simulink model "DVS2X_All"  (R2021b)
settings: Solver=VariableStepAuto  StartTime=0.0  StopTime=0.1  RelTol=1e-3
values from neighbouring files (symbols this model uses):
  k1 = 10^(gain/10)    (= 3.16227766017)    [LNA_tests.m]
  k3 = -4/3*(k1/vip3^2)    [LNA_tests.m]
  k5 = -(0.10875*k1+(3/4)*(vp1dB^2))*((8/5)*(1/vp1dB^4))    [LNA_tests.m]
  vip3 = sqrt(2*10^((IIP3-30)/10)*R)    [LNA_tests.m]
undefined symbols (not defined in the file or in its folder): dvbsapskmod
libraries: commutil2 x23, commdigbbndapm x20, dspsrcs4 x20, commfilt2 x20, commrflib2 x14, commchan3 x12, commsink2 x10, commrandsrc3 x10, commrfcorlib x7, commeq3 x5
(part 1 of 2)
settings Model: SimulationMode=accelerator  Creator=Martha Ca$h  LastModifiedBy=Martha Ca$h
settings SolverCC: AlgebraicLoopSolver=TrustRegion
settings DebuggingCC: SFMachineParentedDataDiag=warning

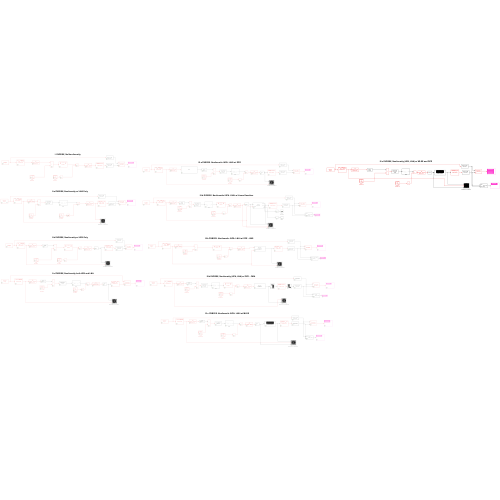
[thumbnail: Simulink's stored preview of the top-level diagram]
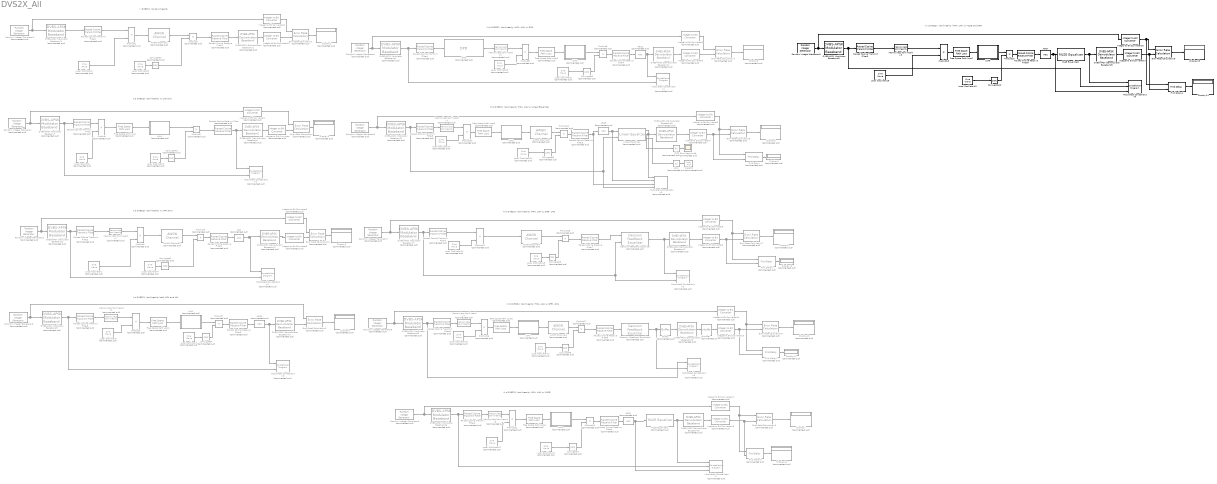
== system DVS2X_All ==
  note: I. DVB2SX, No Non-linearity
  note: II.a DVB2SX, Nonlinearity w/ LNA Only
  note: II.b DVB2SX, Nonlinearity w/ HPA Only
  note: Av
  note: II.c DVB2SX, Nonlinearity both HPA and LNA
  note: III.a DVB2SX, Nonlinearity (HPA, LNA) w/ DPD
  note: III.b DVB2SX, Nonlinearity (HPA, LNA) w/ Linear Equalizer
  note: III.c DVB2SX, Nonlinearity (HPA, LNA) w/ MLSE
  note: III.b DVB2SX, Nonlinearity (HPA, LNA) w/ DFE - LMS
  note: III.b DVB2SX, Nonlinearity (HPA, LNA) w/ DFE - CMA
  note: III.c DVB2SX, Nonlinearity (HPA, LNA) w/ MLSE and DPD
  AGC{,1..4} (5 alike) : commrfcorlib/AGC  Commented=on  LegacyMode=off  DetectorMethod=Rectifier  LoopMethod=Linear  UpdatePeriod=100  StepSize=0.1  AdaptationStepSize=0.01  DesiredOutputPower=1  AveragingLength=256  MaximumGain=30  MaxPowerGain=400  GainOutputPort=off  InputPowerOutputPort=off  SimulateUsing=Code generation
  AGC7 : commrfcorlib/AGC  LegacyMode=off  DetectorMethod=Rectifier  LoopMethod=Linear  UpdatePeriod=100  StepSize=0.1  AdaptationStepSize=0.01  DesiredOutputPower=1  AveragingLength=256  MaximumGain=30  MaxPowerGain=400  GainOutputPort=off  InputPowerOutputPort=off  SimulateUsing=Code generation
  AWGN Channel1 : commchan3/AWGN Channel  Commented=on  InputProcessing=Columns as channels (frame based)  seed=67  noiseMode="Signal to noise ratio  (Eb/No)"  EbNodB=0  EsNodB=10  SNRdB=10  bitsPerSym=4  Ps=1  Tsym=1e-6  variance=1
  AWGN Channel2 : commchan3/AWGN Channel  Commented=on  InputProcessing=Columns as channels (frame based)  seed=67  noiseMode="Signal to noise ratio  (Eb/No)"  EbNodB=23  EsNodB=10  SNRdB=10  bitsPerSym=4  Ps=1  Tsym=1e-6  variance=1
  AWGN Channel3 : commchan3/AWGN Channel  Commented=on  InputProcessing=Columns as channels (frame based)  seed=67  noiseMode="Signal to noise ratio  (Eb/No)"  EbNodB=50  EsNodB=10  SNRdB=10  bitsPerSym=4  Ps=1  Tsym=1e-6  variance=1
  AWGN Channel4 : commchan3/AWGN Channel  Commented=on  InputProcessing=Columns as channels (frame based)  seed=67  noiseMode="Signal to noise ratio  (Eb/No)"  EbNodB=23  EsNodB=10  SNRdB=10  bitsPerSym=4  Ps=1  Tsym=1e-6  variance=1
  AWGN Channel5 : commchan3/AWGN Channel  Commented=on  InputProcessing=Columns as channels (frame based)  seed=67  noiseMode="Signal to noise ratio  (Eb/No)"  EbNodB=23  EsNodB=10  SNRdB=10  bitsPerSym=4  Ps=1  Tsym=1e-6  variance=1
  Abs1 : Abs  Commented=on
  Abs2 : Abs  Commented=on
  Buffer : Buffer  Commented=on  N=16  OutputFrames=off
  Conjugate{1..9} (9 alike) : Math  Commented=on  Operator=conj  SignedPower=on  SaturateOnIntegerOverflow=on
  Conjugate10 : Math  Operator=conj  SignedPower=on  SaturateOnIntegerOverflow=on
  DPD : commrfcorlib/DPD  Commented=on  PolynomialType=Memory polynomial  CoefficientSource=Property  Coefficients=complex([1 0 0 0 0; 0 0 0 0 0; 0 0 0 0 0])  SimulateUsing=Code generation
      settings: SourceProductBaseCode=CM
  DVBS-APSK Demodulator Baseband{,1..8} (9 alike) : commdigbbndapm/DVBS-APSK Demodulator Baseband  Commented=on  StdSuffix=S2  FrameLength=Normal  ModOrder=16  CodeIDF=2/3  NormalizationMethod=Outer radius as 1  OutputType=Integer  DecisionType=Hard decision  VarianceSource=Property  NoiseVariance=1  OutputDataType=double  SimulateUsing=Interpreted execution
      settings: SourceProductBaseCode=CM
  DVBS-APSK Demodulator Baseband9 : commdigbbndapm/DVBS-APSK Demodulator Baseband  StdSuffix=S2  FrameLength=Normal  ModOrder=16  CodeIDF=2/3  NormalizationMethod=Outer radius as 1  OutputType=Integer  DecisionType=Hard decision  VarianceSource=Property  NoiseVariance=1  OutputDataType=double  SimulateUsing=Interpreted execution
      settings: SourceProductBaseCode=CM
  DVBS-APSK Modulator Baseband{,1..8} (9 alike) : commdigbbndapm/DVBS-APSK Modulator Baseband  Commented=on  StdSuffix=S2  FrameLength=Normal  ModOrder=16  CodeIDF=2/3  NormalizationMethod=Outer radius as 1  InputType=Integer  OutputDataType=double  SimulateUsing=Code generation
      settings: SourceProductBaseCode=CM
  DVBS-APSK Modulator Baseband9 : commdigbbndapm/DVBS-APSK Modulator Baseband  StdSuffix=S2  FrameLength=Normal  ModOrder=16  CodeIDF=2/3  NormalizationMethod=Outer radius as 1  InputType=Integer  OutputDataType=double  SimulateUsing=Code generation
      settings: SourceProductBaseCode=CM
  Decision Feedback Equalizer : commeq3/Decision Feedback Equalizer  Commented=on  NumForwardTaps=5  NumFeedbackTaps=3  Constellation=dvbsapskmod(0:15, 16, 's2', '2/3')  InputSamplesPerSymbol=1  Algorithm=LMS  StepSize=0.01  ForgettingFactor=0.99  InitialInverseCorrelationMatrix=0.1  ReferenceTap=3  InputDelay=0  AdaptWeightsSource=Property  AdaptWeights=on  InitialWeightsSource=Auto  InitialWeights=0  TrainingInitialWeights=0  BlindInitialWeights=[ 0; 0; 1; 0; 0; 0; 0; 0 ]  WeightUpdatePeriod=1  TrainingFlagInputPort=off  AdaptAfterTraining=on  ResetInputPort=off  ErrorOutputPort=off  TapWeightsOutputPort=off  SimulateUsing=Code generation
      settings: SourceProductBaseCode=CM
  Decision Feedback Equalizer1 : commeq3/Decision Feedback Equalizer  Commented=on  NumForwardTaps=5  NumFeedbackTaps=3  Constellation=dvbsapskmod(0:15, 16, 's2', '2/3')  InputSamplesPerSymbol=1  Algorithm=CMA  StepSize=0.01  ForgettingFactor=0.99  InitialInverseCorrelationMatrix=0.1  ReferenceTap=3  InputDelay=0  AdaptWeightsSource=Property  AdaptWeights=on  InitialWeightsSource=Auto  InitialWeights=0  TrainingInitialWeights=0  BlindInitialWeights=[ 0; 0; 1; 0; 0; 0; 0; 0 ]  WeightUpdatePeriod=1  TrainingFlagInputPort=off  AdaptAfterTraining=on  ResetInputPort=off  ErrorOutputPort=off  TapWeightsOutputPort=off  SimulateUsing=Code generation
      settings: SourceProductBaseCode=CM
  Display{1..13} (13 alike) : Display  Commented=on
  Display14 : Display
  Display15 : Display
  Error Magnitude : Scope  Commented=on
  Error Rate Calculation : commsink2/Error Rate Calculation  Commented=on  N=40  st_delay=150  cp_mode=Entire frame  subframe=[]  PMode=Port  WsName=ErrorVec1  RsMode2=off  stop=off  numErr=100  maxBits=1e6
  Error Rate Calculation1 : commsink2/Error Rate Calculation  Commented=on  N=40  st_delay=0  cp_mode=Entire frame  subframe=[]  PMode=Port  WsName=ErrorVec1  RsMode2=off  stop=off  numErr=100  maxBits=1e6
  Error Rate Calculation2 : commsink2/Error Rate Calculation  Commented=on  N=40  st_delay=0  cp_mode=Entire frame  subframe=[]  PMode=Port  WsName=ErrorVec1  RsMode2=off  stop=off  numErr=100  maxBits=1e6
  Error Rate Calculation3 : commsink2/Error Rate Calculation  Commented=on  N=10  st_delay=0  cp_mode=Entire frame  subframe=[]  PMode=Port  WsName=ErrorVec1  RsMode2=off  stop=off  numErr=100  maxBits=1e6
  Error Rate Calculation4 : commsink2/Error Rate Calculation  Commented=on  N=40  st_delay=0  cp_mode=Entire frame  subframe=[]  PMode=Port  WsName=ErrorVec1  RsMode2=off  stop=off  numErr=100  maxBits=1e6
  Error Rate Calculation5 : commsink2/Error Rate Calculation  Commented=on  N=40  st_delay=10000  cp_mode=Entire frame  subframe=[]  PMode=Port  WsName=ErrorVec1  RsMode2=off  stop=off  numErr=100  maxBits=1e6
  Error Rate Calculation6 : commsink2/Error Rate Calculation  Commented=on  N=80  st_delay=0  cp_mode=Entire frame  subframe=[]  PMode=Port  WsName=ErrorVec1  RsMode2=off  stop=off  numErr=100  maxBits=1e6
  Error Rate Calculation7 : commsink2/Error Rate Calculation  Commented=on  N=53  st_delay=10000  cp_mode=Entire frame  subframe=[]  PMode=Port  WsName=ErrorVec1  RsMode2=off  stop=off  numErr=100  maxBits=1e6
  Error Rate Calculation8 : commsink2/Error Rate Calculation  Commented=on  N=40  st_delay=10000  cp_mode=Entire frame  subframe=[]  PMode=Port  WsName=ErrorVec1  RsMode2=off  stop=off  numErr=100  maxBits=1e6
  Error Rate Calculation9 : commsink2/Error Rate Calculation  N=80  st_delay=400  cp_mode=Entire frame  subframe=[]  PMode=Port  WsName=ErrorVec1  RsMode2=off  stop=off  numErr=100  maxBits=1e6
  Find Delay : commutil2/Find Delay  Commented=on  corrLength=10000  chgSigOP=off  stopUpdate=off  numConstDelay=3
      settings: SourceProductBaseCode=CM
  Find Delay1 : commutil2/Find Delay  Commented=on  corrLength=10000  chgSigOP=off  stopUpdate=off  numConstDelay=3
      settings: SourceProductBaseCode=CM
  Find Delay2 : commutil2/Find Delay  Commented=on  corrLength=10000  chgSigOP=off  stopUpdate=off  numConstDelay=3
      settings: SourceProductBaseCode=CM
  Find Delay3 : commutil2/Find Delay  Commented=on  corrLength=1000  chgSigOP=off  stopUpdate=off  numConstDelay=3
      settings: SourceProductBaseCode=CM
  Find Delay4 : commutil2/Find Delay  corrLength=1000  chgSigOP=off  stopUpdate=off  numConstDelay=3
      settings: SourceProductBaseCode=CM
  Free Space Path Loss{,1..4,6} (6 alike) : commrflib2/Free Space Path Loss  Commented=on  mode=Decibels  dB=10  d=0.100  fc=1920
      settings: SourceProductBaseCode=CM
  Free Space Path Loss7 : commrflib2/Free Space Path Loss  mode=Decibels  dB=10  d=0.100  fc=1920
      settings: SourceProductBaseCode=CM
  Integer to Bit Converter{,1..15} (16 alike) : commutil2/Integer to Bit Converter  Commented=on  nbits=4  signedInputValues=Unsigned  bitOrder=MSB first  outDtype=Inherit via internal rule
  Integer to Bit Converter16 : commutil2/Integer to Bit Converter  nbits=4  signedInputValues=Unsigned  bitOrder=MSB first  outDtype=Inherit via internal rule
  Integer to Bit Converter17 : commutil2/Integer to Bit Converter  nbits=4  signedInputValues=Unsigned  bitOrder=MSB first  outDtype=Inherit via internal rule
  LNA1 : Subsystem  Commented=on
  LNA2 : Subsystem  Commented=on
  LNA3 : Subsystem  Commented=on
  LNA4 : Subsystem  Commented=on
  LNA5 : Subsystem  Commented=on
  LNA7 : Subsystem  Commented=on
  LNA8 : Subsystem
  Linear Equalizer : commeq3/Linear Equalizer  Commented=on  NumTaps=5  Constellation=dvbsapskmod(0:15, 16, 's2', '2/3')  InputSamplesPerSymbol=1  Algorithm=LMS  StepSize=0.01  ForgettingFactor=0.99  InitialInverseCorrelationMatrix=0.1  ReferenceTap=3  InputDelay=0  AdaptWeightsSource=Property  AdaptWeights=on  InitialWeightsSource=Auto  InitialWeights=0  TrainingInitialWeights=0  BlindInitialWeights=[ 0; 0; 1; 0; 0 ]  WeightUpdatePeriod=1  TrainingFlagInputPort=off  AdaptAfterTraining=on  ResetInputPort=off  ErrorOutputPort=on  TapWeightsOutputPort=on  SimulateUsing=Interpreted execution
      settings: SourceProductBaseCode=CM
  Local Oscillator{,1..17} (18 alike) : dspsrcs4/Sine Wave  Commented=on  Amplitude=1  Frequency=1.5e9  Phase=0  SampleMode=Discrete  OutComplex=Complex  CompMethod=Trigonometric fcn  TableSize=Speed  SampleTime=(1e-6)/8  SamplesPerFrame=8  ResetState=Restart at time zero  OutputFrames=off  dataType=double  wordLen=16  udDataType=sfix(16)  fracBitsMode=Best precision  numFracBits=15  OutDataTypeStr=double  LastOutDataTypeStr=double
  Local Oscillator18 : dspsrcs4/Sine Wave  Amplitude=1  Frequency=1.5e9  Phase=0  SampleMode=Discrete  OutComplex=Complex  CompMethod=Trigonometric fcn  TableSize=Speed  SampleTime=(1e-6)/8  SamplesPerFrame=8  ResetState=Restart at time zero  OutputFrames=off  dataType=double  wordLen=16  udDataType=sfix(16)  fracBitsMode=Best precision  numFracBits=15  OutDataTypeStr=double  LastOutDataTypeStr=double
  Local Oscillator19 : dspsrcs4/Sine Wave  Amplitude=1  Frequency=1.5e9  Phase=0  SampleMode=Discrete  OutComplex=Complex  CompMethod=Trigonometric fcn  TableSize=Speed  SampleTime=(1e-6)/8  SamplesPerFrame=8  ResetState=Restart at time zero  OutputFrames=off  dataType=double  wordLen=16  udDataType=sfix(16)  fracBitsMode=Best precision  numFracBits=15  OutDataTypeStr=double  LastOutDataTypeStr=double
  MLSE Equalizer1 : commeq3/MLSE Equalizer  Commented=on  specchan=Dialog  chancoeff=1  constpts=dvbsapskmod(0:15, 16, 's2', '2/3')  tbdepth=10  opmode=Continuous with reset option  enpreamble=off  preamble=[0 3 2 1]  enpostamble=off  postamble=[0 2 3 1]  numsamp=1  reset=off
      settings: SourceProductBaseCode=CM
  MLSE Equalizer2 : commeq3/MLSE Equalizer  specchan=Dialog  chancoeff=1  constpts=dvbsapskmod(0:15, 16, 's2', '2/3')  tbdepth=10  opmode=Continuous with reset option  enpreamble=off  preamble=[0 3 2 1]  enpostamble=off  postamble=[0 2 3 1]  numsamp=1  reset=off
      settings: SourceProductBaseCode=CM
  Memoryless Nonlinearity1 : commrflib2/Memoryless Nonlinearity  Commented=on  model_select=Saleh model  linGaindB=0  GindB=GindB  iip3=30  am2pm=10  LPwrLimAMPM=10  UPwrLimAMPM=inf  amam=[2.1587 1.1517]  ampm=[4.0330 9.1040]  x=[8.1081 1.5413 6.5202 -0.0718]  y=[4.6645 2.0965 10.88 -0.003]  p=0.5  GoutdB=GoutdB  vsat=1
      settings: SourceProductBaseCode=CM
  Memoryless Nonlinearity2 : commrflib2/Memoryless Nonlinearity  Commented=on  model_select=Saleh model  linGaindB=0  GindB=GindB  iip3=30  am2pm=10  LPwrLimAMPM=10  UPwrLimAMPM=inf  amam=[2.1587 1.1517]  ampm=[4.0330 9.1040]  x=[8.1081 1.5413 6.5202 -0.0718]  y=[4.6645 2.0965 10.88 -0.003]  p=0.5  GoutdB=GoutdB  vsat=1
      settings: SourceProductBaseCode=CM
  Memoryless Nonlinearity3 : commrflib2/Memoryless Nonlinearity  Commented=on  model_select=Saleh model  linGaindB=0  GindB=GindB  iip3=30  am2pm=10  LPwrLimAMPM=10  UPwrLimAMPM=inf  amam=[2.1587 1.1517]  ampm=[4.0330 9.1040]  x=[8.1081 1.5413 6.5202 -0.0718]  y=[4.6645 2.0965 10.88 -0.003]  p=0.5  GoutdB=GoutdB  vsat=1
      settings: SourceProductBaseCode=CM
  Memoryless Nonlinearity4 : commrflib2/Memoryless Nonlinearity  Commented=on  model_select=Saleh model  linGaindB=0  GindB=-7.626571802255640  iip3=30  am2pm=10  LPwrLimAMPM=10  UPwrLimAMPM=inf  amam=[2.1587 1.1517]  ampm=[4.0330 9.1040]  x=[8.1081 1.5413 6.5202 -0.0718]  y=[4.6645 2.0965 10.88 -0.003]  p=0.5  GoutdB=9.911826101838730  vsat=1
      settings: SourceProductBaseCode=CM
  Memoryless Nonlinearity5 : commrflib2/Memoryless Nonlinearity  Commented=on  model_select=Saleh model  linGaindB=0  GindB=-7.626571802255640  iip3=30  am2pm=10  LPwrLimAMPM=10  UPwrLimAMPM=inf  amam=[2.1587 1.1517]  ampm=[4.0330 9.1040]  x=[8.1081 1.5413 6.5202 -0.0718]  y=[4.6645 2.0965 10.88 -0.003]  p=0.5  GoutdB=9.911826101838730  vsat=1
      settings: SourceProductBaseCode=CM
  Memoryless Nonlinearity7 : commrflib2/Memoryless Nonlinearity  Commented=on  model_select=Saleh model  linGaindB=0  GindB=-7.626571802255640  iip3=30  am2pm=10  LPwrLimAMPM=10  UPwrLimAMPM=inf  amam=[2.1587 1.1517]  ampm=[4.0330 9.1040]  x=[8.1081 1.5413 6.5202 -0.0718]  y=[4.6645 2.0965 10.88 -0.003]  p=0.5  GoutdB=9.911826101838730  vsat=1
      settings: SourceProductBaseCode=CM
  Memoryless Nonlinearity8 : commrflib2/Memoryless Nonlinearity  model_select=Saleh model  linGaindB=0  GindB=-7.626571802255640  iip3=30  am2pm=10  LPwrLimAMPM=10  UPwrLimAMPM=inf  amam=[2.1587 1.1517]  ampm=[4.0330 9.1040]  x=[8.1081 1.5413 6.5202 -0.0718]  y=[4.6645 2.0965 10.88 -0.003]  p=0.5  GoutdB=9.911826101838730  vsat=1
      settings: SourceProductBaseCode=CM
  Modulated Constellation{1..4,6,8} (6 alike) : ConstellationDiagram  Commented=on  NumInputPorts=2
  Modulated Constellation5 : ConstellationDiagram  Commented=on  NumInputPorts=4
  Modulated Constellation7 : ConstellationDiagram  Commented=on  NumInputPorts=3
  Modulated Constellation9 : ConstellationDiagram  NumInputPorts=3
  Product{,1..17} (18 alike) : Product  Commented=on
  Product18 : Product
  Product19 : Product
  Raised Cosine Receive Filter : commfilt2/Raised Cosine Receive Filter  Commented=on  filtType=Square root  R=0.2  filtSpan=10  N=8  downFactor=8  downOffset=0  filterGain=1  InputProcessing=Columns as channels (frame based)  RateOptions=Enforce single-rate processing  framing=Mute  checkCoeff=off  variableName=rcRxFilt  currentFiltSpan=10  D=(10)/2  inputOffset=0  sampMode=Mute  saveAsFlag=0  rateMode=Downsampling  checkGain=Normalized  launchFVT=on  roundingMode=Floor  overflowMode=off  coeffDataTypeStr=Inherit: Same word length as input  coeffMin=[]  coeffMax=[]  coeffLastDataTypeStr=Inherit: Same word length as input  accumDataTypeStr=Inherit: Same as product output  accumLastDataTypeStr=Inherit: Same as product output  outputDataTypeStr=Inherit: Same as accumulator  outputMin=[]  outputMax=[]  outputLastDataTypeStr=Inherit: Same as accumulator
  Raised Cosine Receive Filter1 : commfilt2/Raised Cosine Receive Filter  Commented=on  filtType=Square root  R=0.2  filtSpan=10  N=8  downFactor=8  downOffset=0  filterGain=1  InputProcessing=Columns as channels (frame based)  RateOptions=Enforce single-rate processing  framing=Mute  checkCoeff=off  variableName=rcRxFilt1  currentFiltSpan=10  D=(10)/2  inputOffset=0  sampMode=Mute  saveAsFlag=0  rateMode=Downsampling  checkGain=Normalized  launchFVT=on  roundingMode=Floor  overflowMode=off  coeffDataTypeStr=Inherit: Same word length as input  coeffMin=[]  coeffMax=[]  coeffLastDataTypeStr=Inherit: Same word length as input  accumDataTypeStr=Inherit: Same as product output  accumLastDataTypeStr=Inherit: Same as product output  outputDataTypeStr=Inherit: Same as accumulator  outputMin=[]  outputMax=[]  outputLastDataTypeStr=Inherit: Same as accumulator
  Raised Cosine Receive Filter2 : commfilt2/Raised Cosine Receive Filter  Commented=on  filtType=Square root  R=0.2  filtSpan=10  N=8  downFactor=8  downOffset=0  filterGain=1  InputProcessing=Columns as channels (frame based)  RateOptions=Enforce single-rate processing  framing=Mute  checkCoeff=off  variableName=rcRxFilt2  currentFiltSpan=10  D=(10)/2  inputOffset=0  sampMode=Mute  saveAsFlag=0  rateMode=Downsampling  checkGain=Normalized  launchFVT=on  roundingMode=Floor  overflowMode=off  coeffDataTypeStr=Inherit: Same word length as input  coeffMin=[]  coeffMax=[]  coeffLastDataTypeStr=Inherit: Same word length as input  accumDataTypeStr=Inherit: Same as product output  accumLastDataTypeStr=Inherit: Same as product output  outputDataTypeStr=Inherit: Same as accumulator  outputMin=[]  outputMax=[]  outputLastDataTypeStr=Inherit: Same as accumulator
  Raised Cosine Receive Filter3 : commfilt2/Raised Cosine Receive Filter  Commented=on  filtType=Square root  R=0.2  filtSpan=10  N=8  downFactor=8  downOffset=0  filterGain=1  InputProcessing=Columns as channels (frame based)  RateOptions=Enforce single-rate processing  framing=Mute  checkCoeff=off  variableName=rcRxFilt3  currentFiltSpan=10  D=(10)/2  inputOffset=0  sampMode=Mute  saveAsFlag=0  rateMode=Downsampling  checkGain=Normalized  launchFVT=on  roundingMode=Floor  overflowMode=off  coeffDataTypeStr=Inherit: Same word length as input  coeffMin=[]  coeffMax=[]  coeffLastDataTypeStr=Inherit: Same word length as input  accumDataTypeStr=Inherit: Same as product output  accumLastDataTypeStr=Inherit: Same as product output  outputDataTypeStr=Inherit: Same as accumulator  outputMin=[]  outputMax=[]  outputLastDataTypeStr=Inherit: Same as accumulator
  Raised Cosine Receive Filter4 : commfilt2/Raised Cosine Receive Filter  Commented=on  filtType=Square root  R=0.2  filtSpan=10  N=8  downFactor=8  downOffset=0  filterGain=1  InputProcessing=Columns as channels (frame based)  RateOptions=Enforce single-rate processing  framing=Mute  checkCoeff=off  variableName=rcRxFilt4  currentFiltSpan=10  D=(10)/2  inputOffset=0  sampMode=Mute  saveAsFlag=0  rateMode=Downsampling  checkGain=Normalized  launchFVT=on  roundingMode=Floor  overflowMode=off  coeffDataTypeStr=Inherit: Same word length as input  coeffMin=[]  coeffMax=[]  coeffLastDataTypeStr=Inherit: Same word length as input  accumDataTypeStr=Inherit: Same as product output  accumLastDataTypeStr=Inherit: Same as product output  outputDataTypeStr=Inherit: Same as accumulator  outputMin=[]  outputMax=[]  outputLastDataTypeStr=Inherit: Same as accumulator
  Raised Cosine Receive Filter5 : commfilt2/Raised Cosine Receive Filter  Commented=on  filtType=Square root  R=0.2  filtSpan=10  N=8  downFactor=8  downOffset=0  filterGain=1  InputProcessing=Columns as channels (frame based)  RateOptions=Enforce single-rate processing  framing=Mute  checkCoeff=off  variableName=rcRxFilt5  currentFiltSpan=10  D=(10)/2  inputOffset=0  sampMode=Mute  saveAsFlag=0  rateMode=Downsampling  checkGain=Normalized  launchFVT=on  roundingMode=Floor  overflowMode=off  coeffDataTypeStr=Inherit: Same word length as input  coeffMin=[]  coeffMax=[]  coeffLastDataTypeStr=Inherit: Same word length as input  accumDataTypeStr=Inherit: Same as product output  accumLastDataTypeStr=Inherit: Same as product output  outputDataTypeStr=Inherit: Same as accumulator  outputMin=[]  outputMax=[]  outputLastDataTypeStr=Inherit: Same as accumulator
  Raised Cosine Receive Filter6 : commfilt2/Raised Cosine Receive Filter  Commented=on  filtType=Square root  R=0.2  filtSpan=10  N=8  downFactor=8  downOffset=0  filterGain=1  InputProcessing=Columns as channels (frame based)  RateOptions=Enforce single-rate processing  framing=Mute  checkCoeff=off  variableName=rcRxFilt6  currentFiltSpan=10  D=(10)/2  inputOffset=0  sampMode=Mute  saveAsFlag=0  rateMode=Downsampling  checkGain=Normalized  launchFVT=on  roundingMode=Floor  overflowMode=off  coeffDataTypeStr=Inherit: Same word length as input  coeffMin=[]  coeffMax=[]  coeffLastDataTypeStr=Inherit: Same word length as input  accumDataTypeStr=Inherit: Same as product output  accumLastDataTypeStr=Inherit: Same as product output  outputDataTypeStr=Inherit: Same as accumulator  outputMin=[]  outputMax=[]  outputLastDataTypeStr=Inherit: Same as accumulator
  Raised Cosine Receive Filter7 : commfilt2/Raised Cosine Receive Filter  Commented=on  filtType=Square root  R=0.2  filtSpan=10  N=8  downFactor=8  downOffset=0  filterGain=1  InputProcessing=Columns as channels (frame based)  RateOptions=Enforce single-rate processing  framing=Mute  checkCoeff=off  variableName=rcRxFilt7  currentFiltSpan=10  D=(10)/2  inputOffset=0  sampMode=Mute  saveAsFlag=0  rateMode=Downsampling  checkGain=Normalized  launchFVT=on  roundingMode=Floor  overflowMode=off  coeffDataTypeStr=Inherit: Same word length as input  coeffMin=[]  coeffMax=[]  coeffLastDataTypeStr=Inherit: Same word length as input  accumDataTypeStr=Inherit: Same as product output  accumLastDataTypeStr=Inherit: Same as product output  outputDataTypeStr=Inherit: Same as accumulator  outputMin=[]  outputMax=[]  outputLastDataTypeStr=Inherit: Same as accumulator
  Raised Cosine Receive Filter8 : commfilt2/Raised Cosine Receive Filter  Commented=on  filtType=Square root  R=0.2  filtSpan=10  N=8  downFactor=8  downOffset=0  filterGain=1  InputProcessing=Columns as channels (frame based)  RateOptions=Enforce single-rate processing  framing=Mute  checkCoeff=off  variableName=rcRxFilt8  currentFiltSpan=10  D=(10)/2  inputOffset=0  sampMode=Mute  saveAsFlag=0  rateMode=Downsampling  checkGain=Normalized  launchFVT=on  roundingMode=Floor  overflowMode=off  coeffDataTypeStr=Inherit: Same word length as input  coeffMin=[]  coeffMax=[]  coeffLastDataTypeStr=Inherit: Same word length as input  accumDataTypeStr=Inherit: Same as product output  accumLastDataTypeStr=Inherit: Same as product output  outputDataTypeStr=Inherit: Same as accumulator  outputMin=[]  outputMax=[]  outputLastDataTypeStr=Inherit: Same as accumulator
  Raised Cosine Receive Filter9 : commfilt2/Raised Cosine Receive Filter  filtType=Square root  R=0.2  filtSpan=10  N=8  downFactor=8  downOffset=0  filterGain=1  InputProcessing=Columns as channels (frame based)  RateOptions=Enforce single-rate processing  framing=Mute  checkCoeff=off  variableName=rcRxFilt9  currentFiltSpan=10  D=(10)/2  inputOffset=0  sampMode=Mute  saveAsFlag=0  rateMode=Downsampling  checkGain=Normalized  launchFVT=on  roundingMode=Floor  overflowMode=off  coeffDataTypeStr=Inherit: Same word length as input  coeffMin=[]  coeffMax=[]  coeffLastDataTypeStr=Inherit: Same word length as input  accumDataTypeStr=Inherit: Same as product output  accumLastDataTypeStr=Inherit: Same as product output  outputDataTypeStr=Inherit: Same as accumulator  outputMin=[]  outputMax=[]  outputLastDataTypeStr=Inherit: Same as accumulator
  Raised Cosine Transmit Filter : commfilt2/Raised Cosine Transmit Filter  Commented=on  filtType=Square root  R=0.2  filtSpan=10  N=8  filterGain=1  InputProcessing=Columns as channels (frame based)  RateOptions=Enforce single-rate processing  framing=Mute  checkCoeff=on  variableName=rcTxFilt  checkGain=Normalized  sampMode=Mute  saveAsFlag=0  currentFiltSpan=10  D=(10)/2  launchFVT=on  roundingMode=Floor  overflowMode=off  coeffDataTypeStr=Inherit: Same word length as input  coeffMin=[]  coeffMax=[]  coeffLastDataTypeStr=Inherit: Same word length as input  outputDataTypeStr=Inherit: Same as accumulator  outputMin=[]  outputMax=[]  outputLastDataTypeStr=Inherit: Same as accumulator
  Raised Cosine Transmit Filter1 : commfilt2/Raised Cosine Transmit Filter  Commented=on  filtType=Square root  R=0.2  filtSpan=10  N=8  filterGain=1  InputProcessing=Columns as channels (frame based)  RateOptions=Enforce single-rate processing  framing=Mute  checkCoeff=on  variableName=rcTxFilt1  checkGain=Normalized  sampMode=Mute  saveAsFlag=0  currentFiltSpan=10  D=(10)/2  launchFVT=on  roundingMode=Floor  overflowMode=off  coeffDataTypeStr=Inherit: Same word length as input  coeffMin=[]  coeffMax=[]  coeffLastDataTypeStr=Inherit: Same word length as input  outputDataTypeStr=Inherit: Same as accumulator  outputMin=[]  outputMax=[]  outputLastDataTypeStr=Inherit: Same as accumulator
  Raised Cosine Transmit Filter2 : commfilt2/Raised Cosine Transmit Filter  Commented=on  filtType=Square root  R=0.2  filtSpan=10  N=8  filterGain=1  InputProcessing=Columns as channels (frame based)  RateOptions=Enforce single-rate processing  framing=Mute  checkCoeff=on  variableName=rcTxFilt2  checkGain=Normalized  sampMode=Mute  saveAsFlag=0  currentFiltSpan=10  D=(10)/2  launchFVT=on  roundingMode=Floor  overflowMode=off  coeffDataTypeStr=Inherit: Same word length as input  coeffMin=[]  coeffMax=[]  coeffLastDataTypeStr=Inherit: Same word length as input  outputDataTypeStr=Inherit: Same as accumulator  outputMin=[]  outputMax=[]  outputLastDataTypeStr=Inherit: Same as accumulator
  Raised Cosine Transmit Filter3 : commfilt2/Raised Cosine Transmit Filter  Commented=on  filtType=Square root  R=0.2  filtSpan=10  N=8  filterGain=1  InputProcessing=Columns as channels (frame based)  RateOptions=Enforce single-rate processing  framing=Mute  checkCoeff=on  variableName=rcTxFilt3  checkGain=Normalized  sampMode=Mute  saveAsFlag=0  currentFiltSpan=10  D=(10)/2  launchFVT=on  roundingMode=Floor  overflowMode=off  coeffDataTypeStr=Inherit: Same word length as input  coeffMin=[]  coeffMax=[]  coeffLastDataTypeStr=Inherit: Same word length as input  outputDataTypeStr=Inherit: Same as accumulator  outputMin=[]  outputMax=[]  outputLastDataTypeStr=Inherit: Same as accumulator
  Raised Cosine Transmit Filter4 : commfilt2/Raised Cosine Transmit Filter  Commented=on  filtType=Square root  R=0.2  filtSpan=10  N=8  filterGain=1  InputProcessing=Columns as channels (frame based)  RateOptions=Enforce single-rate processing  framing=Mute  checkCoeff=on  variableName=rcTxFilt4  checkGain=Normalized  sampMode=Mute  saveAsFlag=0  currentFiltSpan=10  D=(10)/2  launchFVT=on  roundingMode=Floor  overflowMode=off  coeffDataTypeStr=Inherit: Same word length as input  coeffMin=[]  coeffMax=[]  coeffLastDataTypeStr=Inherit: Same word length as input  outputDataTypeStr=Inherit: Same as accumulator  outputMin=[]  outputMax=[]  outputLastDataTypeStr=Inherit: Same as accumulator
  Raised Cosine Transmit Filter5 : commfilt2/Raised Cosine Transmit Filter  Commented=on  filtType=Square root  R=0.2  filtSpan=10  N=8  filterGain=1  InputProcessing=Columns as channels (frame based)  RateOptions=Enforce single-rate processing  framing=Mute  checkCoeff=on  variableName=rcTxFilt5  checkGain=Normalized  sampMode=Mute  saveAsFlag=0  currentFiltSpan=10  D=(10)/2  launchFVT=on  roundingMode=Floor  overflowMode=off  coeffDataTypeStr=Inherit: Same word length as input  coeffMin=[]  coeffMax=[]  coeffLastDataTypeStr=Inherit: Same word length as input  outputDataTypeStr=Inherit: Same as accumulator  outputMin=[]  outputMax=[]  outputLastDataTypeStr=Inherit: Same as accumulator
  Raised Cosine Transmit Filter6 : commfilt2/Raised Cosine Transmit Filter  Commented=on  filtType=Square root  R=0.2  filtSpan=10  N=8  filterGain=1  InputProcessing=Columns as channels (frame based)  RateOptions=Enforce single-rate processing  framing=Mute  checkCoeff=on  variableName=rcTxFilt6  checkGain=Normalized  sampMode=Mute  saveAsFlag=0  currentFiltSpan=10  D=(10)/2  launchFVT=on  roundingMode=Floor  overflowMode=off  coeffDataTypeStr=Inherit: Same word length as input  coeffMin=[]  coeffMax=[]  coeffLastDataTypeStr=Inherit: Same word length as input  outputDataTypeStr=Inherit: Same as accumulator  outputMin=[]  outputMax=[]  outputLastDataTypeStr=Inherit: Same as accumulator
  Raised Cosine Transmit Filter7 : commfilt2/Raised Cosine Transmit Filter  Commented=on  filtType=Square root  R=0.2  filtSpan=10  N=8  filterGain=1  InputProcessing=Columns as channels (frame based)  RateOptions=Enforce single-rate processing  framing=Mute  checkCoeff=on  variableName=rcTxFilt7  checkGain=Normalized  sampMode=Mute  saveAsFlag=0  currentFiltSpan=10  D=(10)/2  launchFVT=on  roundingMode=Floor  overflowMode=off  coeffDataTypeStr=Inherit: Same word length as input  coeffMin=[]  coeffMax=[]  coeffLastDataTypeStr=Inherit: Same word length as input  outputDataTypeStr=Inherit: Same as accumulator  outputMin=[]  outputMax=[]  outputLastDataTypeStr=Inherit: Same as accumulator
  Raised Cosine Transmit Filter8 : commfilt2/Raised Cosine Transmit Filter  Commented=on  filtType=Square root  R=0.2  filtSpan=10  N=8  filterGain=1  InputProcessing=Columns as channels (frame based)  RateOptions=Enforce single-rate processing  framing=Mute  checkCoeff=on  variableName=rcTxFilt8  checkGain=Normalized  sampMode=Mute  saveAsFlag=0  currentFiltSpan=10  D=(10)/2  launchFVT=on  roundingMode=Floor  overflowMode=off  coeffDataTypeStr=Inherit: Same word length as input  coeffMin=[]  coeffMax=[]  coeffLastDataTypeStr=Inherit: Same word length as input  outputDataTypeStr=Inherit: Same as accumulator  outputMin=[]  outputMax=[]  outputLastDataTypeStr=Inherit: Same as accumulator
  Raised Cosine Transmit Filter9 : commfilt2/Raised Cosine Transmit Filter  filtType=Square root  R=0.2  filtSpan=10  N=8  filterGain=1  InputProcessing=Columns as channels (frame based)  RateOptions=Enforce single-rate processing  framing=Mute  checkCoeff=on  variableName=rcTxFilt9  checkGain=Normalized  sampMode=Mute  saveAsFlag=0  currentFiltSpan=10  D=(10)/2  launchFVT=on  roundingMode=Floor  overflowMode=off  coeffDataTypeStr=Inherit: Same word length as input  coeffMin=[]  coeffMax=[]  coeffLastDataTypeStr=Inherit: Same word length as input  outputDataTypeStr=Inherit: Same as accumulator  outputMin=[]  outputMax=[]  outputLastDataTypeStr=Inherit: Same as accumulator
  Random Integer Generator{,1..8} (9 alike) : commrandsrc3/Random Integer Generator  Commented=on  SetSize=16  SeedSource=Auto  Seed=0  SampleTime=1e-6  SamplesPerFrame=1  OutputDataType=double  SimulateUsing=Interpreted execution
  Random Integer Generator9 : commrandsrc3/Random Integer Generator  SetSize=16  SeedSource=Auto  Seed=0  SampleTime=1e-6  SamplesPerFrame=1  OutputDataType=double  SimulateUsing=Interpreted execution
  Unbuffer : Unbuffer  Commented=on  ic=16
  Weights : ArrayPlot  Commented=on  WindowPosition=[470 203 340 314]  XOffset=1  AxesScaling=Manual  YLimits=[-0.081846,1.76573]  DefaultConfigurationName=dsp.scopes.ArrayPlotBlockSpecification
  wires:
  DVBS-APSK Modulator Baseband1/1 -> Raised Cosine Transmit Filter1/1
  Product3/1 -> Raised Cosine Receive Filter1/1
  AWGN Channel1/1 -> Product3/1
  Local Oscillator2/1 -> Product2/2
  Random Integer Generator1/1 -> DVBS-APSK Modulator Baseband1/1, Integer to Bit Converter11/1
  Product2/1 -> AWGN Channel1/1
  Raised Cosine Transmit Filter1/1 -> Product2/1
  Local Oscillator3/1 -> Conjugate2/1
  Raised Cosine Receive Filter1/1 -> DVBS-APSK Demodulator Baseband1/1
  Error Rate Calculation1/1 -> Display1/1
  Conjugate2/1 -> Product3/2
  DVBS-APSK Demodulator Baseband1/1 -> Integer to Bit Converter10/1
  DVBS-APSK Modulator Baseband2/1 -> Modulated Constellation2/2, Raised Cosine Transmit Filter2/1
  Product4/1 -> Raised Cosine Receive Filter2/1
  AWGN Channel2/1 -> Product4/1
  Local Oscillator1/1 -> Product1/2
  Raised Cosine Transmit Filter2/1 -> Memoryless Nonlinearity1/1
  Random Integer Generator2/1 -> DVBS-APSK Modulator Baseband2/1, Integer to Bit Converter2/1
  Product1/1 -> AWGN Channel2/1
  Memoryless Nonlinearity1/1 -> Product1/1
  Local Oscillator4/1 -> Conjugate1/1
  Error Rate Calculation2/1 -> Display2/1
  Conjugate1/1 -> Product4/2
  DVBS-APSK Demodulator Baseband2/1 -> Integer to Bit Converter3/1
  Raised Cosine Transmit Filter/1 -> Product/1
  LNA4/1("Y ") -> Product5/1
  Product5/1 -> Raised Cosine Receive Filter/1
  Error Rate Calculation/1 -> Display3/1
  Raised Cosine Receive Filter/1 -> Modulated Constellation1/1, DVBS-APSK Demodulator Baseband/1
  DVBS-APSK Demodulator Baseband/1 -> Integer to Bit Converter/1
  Local Oscillator/1 -> Product/2
  Local Oscillator5/1 -> Conjugate3/1
  Product/1 -> Free Space Path Loss/1
  Conjugate3/1 -> Product5/2
  DVBS-APSK Modulator Baseband/1 -> Modulated Constellation1/2, Raised Cosine Transmit Filter/1
  Random Integer Generator/1 -> Integer to Bit Converter1/1, DVBS-APSK Modulator Baseband/1
  Random Integer Generator3/1 -> DVBS-APSK Modulator Baseband3/1, Error Rate Calculation3/1
  Raised Cosine Transmit Filter3/1 -> Memoryless Nonlinearity2/1
  Local Oscillator6/1 -> Product6/2
  DVBS-APSK Modulator Baseband3/1 -> Raised Cosine Transmit Filter3/1, Modulated Constellation3/2
  Memoryless Nonlinearity2/1 -> Product6/1
  Product6/1 -> Free Space Path Loss1/1
  Product7/1 -> Raised Cosine Receive Filter3/1
  Local Oscillator7/1 -> Conjugate4/1
  Raised Cosine Receive Filter3/1 -> AGC1/1
  Conjugate4/1 -> Product7/2
  Error Rate Calculation3/1 -> Display4/1
  DVBS-APSK Demodulator Baseband3/1 -> Error Rate Calculation3/2
  LNA1/1("Y ") -> Product7/1
  Free Space Path Loss1/1 -> LNA1/1("X ")
  Random Integer Generator4/1 -> Integer to Bit Converter4/1, DVBS-APSK Modulator Baseband4/1
  Local Oscillator8/1 -> Product8/2
  Product9/1 -> Raised Cosine Receive Filter4/1
  Local Oscillator9/1 -> Conjugate5/1
  Conjugate5/1 -> Product9/2
  Error Rate Calculation4/1 -> Display5/1
  DVBS-APSK Demodulator Baseband4/1 -> Integer to Bit Converter5/1
  LNA2/1("Y ") -> Product9/1
  Local Oscillator11/1 -> Conjugate6/1
  Memoryless Nonlinearity4/1 -> Product10/1
  Product11/1 -> Raised Cosine Receive Filter5/1
  Error Rate Calculation5/1 -> Display6/1
  Conjugate6/1 -> Product11/2
  AWGN Channel5/1 -> Product11/1
  Product10/1 -> Free Space Path Loss3/1
  Raised Cosine Transmit Filter5/1 -> Memoryless Nonlinearity4/1
  Local Oscillator10/1 -> Product10/2
  LNA3/1("Y ") -> AWGN Channel5/1
  Random Integer Generator5/1 -> DVBS-APSK Modulator Baseband5/1, Integer to Bit Converter6/1
  DVBS-APSK Demodulator Baseband5/1 -> Integer to Bit Converter7/1
  Free Space Path Loss/1 -> LNA4/1("X ")
  Free Space Path Loss2/1 -> LNA2/1("X ")
  Product8/1 -> Free Space Path Loss2/1
  Free Space Path Loss3/1 -> LNA3/1("X ")
  Local Oscillator13/1 -> Conjugate7/1
  Product13/1 -> Raised Cosine Receive Filter6/1
  Free Space Path Loss4/1 -> LNA5/1("X ")
  Error Rate Calculation6/1 -> Display7/1
  Conjugate7/1 -> Product13/2
  DVBS-APSK Modulator Baseband6/1 -> Raised Cosine Transmit Filter6/1, Modulated Constellation7/2
  LNA5/1("Y ") -> Product13/1
  Raised Cosine Transmit Filter6/1 -> Memoryless Nonlinearity5/1
  Random Integer Generator6/1 -> DVBS-APSK Modulator Baseband6/1, Integer to Bit Converter12/1
  Product12/1 -> Free Space Path Loss4/1
  Local Oscillator12/1 -> Product12/2
  DVBS-APSK Modulator Baseband4/1 -> Modulated Constellation4/2, Raised Cosine Transmit Filter4/1
  Memoryless Nonlinearity3/1 -> Product8/1
  Integer to Bit Converter1/1 -> Error Rate Calculation/1
  Integer to Bit Converter/1 -> Error Rate Calculation/2
  Integer to Bit Converter2/1 -> Error Rate Calculation2/1
  Integer to Bit Converter3/1 -> Error Rate Calculation2/2
  AGC/1 -> Modulated Constellation2/1, DVBS-APSK Demodulator Baseband2/1
  Raised Cosine Receive Filter2/1 -> AGC/1
  AGC1/1 -> Modulated Constellation3/1, DVBS-APSK Demodulator Baseband3/1
  Integer to Bit Converter4/1 -> Error Rate Calculation4/1
  Integer to Bit Converter5/1 -> Error Rate Calculation4/2
  AGC2/1 -> Modulated Constellation4/1, DVBS-APSK Demodulator Baseband4/1
  Raised Cosine Receive Filter4/1 -> AGC2/1
  Raised Cosine Transmit Filter4/1 -> DPD/1
  DPD/1 -> Memoryless Nonlinearity3/1
  Integer to Bit Converter6/1 -> Find Delay/1, Error Rate Calculation5/1
  Integer to Bit Converter7/1 -> Find Delay/2, Error Rate Calculation5/2
  Find Delay/1 -> Display8/1
  Linear Equalizer/1 -> Modulated Constellation5/1, DVBS-APSK Demodulator Baseband5/1
  Raised Cosine Receive Filter5/1 -> Modulated Constellation5/3, AGC3/1
  AGC3/1 -> Modulated Constellation5/2, Linear Equalizer/1
  DVBS-APSK Modulator Baseband5/1 -> Raised Cosine Transmit Filter5/1, Linear Equalizer/2, Modulated Constellation5/4
  Abs1/1 -> Weights/1
  Abs2/1 -> Error Magnitude/1
  Linear Equalizer/2 -> Abs2/1
  Linear Equalizer/3 -> Abs1/1
  Integer to Bit Converter8/1 -> Find Delay1/1, Error Rate Calculation7/1
  Error Rate Calculation7/1 -> Display9/1
  DVBS-APSK Demodulator Baseband7/1 -> Integer to Bit Converter9/1
  DVBS-APSK Modulator Baseband7/1 -> Raised Cosine Transmit Filter7/1, Modulated Constellation6/2, Decision Feedback Equalizer/2
  Integer to Bit Converter9/1 -> Find Delay1/2, Error Rate Calculation7/2
  Conjugate8/1 -> Product15/2
  Local Oscillator15/1 -> Conjugate8/1
  Local Oscillator14/1 -> Product14/2
  Product15/1 -> Raised Cosine Receive Filter7/1
  Product14/1 -> AWGN Channel3/1
  Random Integer Generator7/1 -> DVBS-APSK Modulator Baseband7/1, Integer to Bit Converter8/1
  Raised Cosine Transmit Filter7/1 -> Product14/1
  Find Delay1/1 -> Display10/1
  Decision Feedback Equalizer/1 -> Modulated Constellation6/1, DVBS-APSK Demodulator Baseband7/1
  Raised Cosine Receive Filter7/1 -> Decision Feedback Equalizer/1
  Memoryless Nonlinearity5/1 -> Product12/1
  MLSE Equalizer1/1 -> DVBS-APSK Demodulator Baseband6/1, Modulated Constellation7/1
  Integer to Bit Converter11/1 -> Error Rate Calculation1/1
  Integer to Bit Converter10/1 -> Error Rate Calculation1/2
  Integer to Bit Converter12/1 -> Find Delay3/1, Error Rate Calculation6/1
  Find Delay3/1 -> Display12/1
  Product17/1 -> Raised Cosine Receive Filter8/1
  Random Integer Generator8/1 -> DVBS-APSK Modulator Baseband8/1, Integer to Bit Converter14/1
  Free Space Path Loss6/1 -> LNA7/1("X ")
  Memoryless Nonlinearity7/1 -> Product16/1
  Find Delay2/1 -> Display11/1
  LNA7/1("Y ") -> AWGN Channel4/1
  Local Oscillator17/1 -> Conjugate9/1
  Conjugate9/1 -> Product17/2
  Integer to Bit Converter15/1 -> Find Delay2/2, Error Rate Calculation8/2
  Raised Cosine Receive Filter8/1 -> Decision Feedback Equalizer1/1
  Product16/1 -> Free Space Path Loss6/1
  AWGN Channel4/1 -> Product17/1
  Local Oscillator16/1 -> Product16/2
  Error Rate Calculation8/1 -> Display13/1
  DVBS-APSK Modulator Baseband8/1 -> Modulated Constellation8/1, Raised Cosine Transmit Filter8/1
  Integer to Bit Converter14/1 -> Find Delay2/1, Error Rate Calculation8/1
  Raised Cosine Transmit Filter8/1 -> Memoryless Nonlinearity7/1
  Decision Feedback Equalizer1/1 -> Buffer/1, Modulated Constellation8/2
  Buffer/1 -> DVBS-APSK Demodulator Baseband8/1
  DVBS-APSK Demodulator Baseband8/1 -> Unbuffer/1
  Unbuffer/1 -> Integer to Bit Converter15/1
  Find Delay4/1 -> Display14/1
  Integer to Bit Converter17/1 -> Find Delay4/2, Error Rate Calculation9/2
  Integer to Bit Converter16/1 -> Find Delay4/1, Error Rate Calculation9/1
  MLSE Equalizer2/1 -> DVBS-APSK Demodulator Baseband9/1, Modulated Constellation9/1
  Raised Cosine Receive Filter9/1 -> AGC7/1
  Product18/1 -> Free Space Path Loss7/1
  Error Rate Calculation9/1 -> Display15/1
  DVBS-APSK Demodulator Baseband9/1 -> Integer to Bit Converter17/1
  Memoryless Nonlinearity8/1 -> Product18/1
  Product19/1 -> Raised Cosine Receive Filter9/1
  DVBS-APSK Modulator Baseband9/1 -> Raised Cosine Transmit Filter9/1, Modulated Constellation9/2
  LNA8/1("Y ") -> Product19/1
  Random Integer Generator9/1 -> DVBS-APSK Modulator Baseband9/1, Integer to Bit Converter16/1
  Local Oscillator19/1 -> Conjugate10/1
  Conjugate10/1 -> Product19/2
  Free Space Path Loss7/1 -> LNA8/1("X ")
  Local Oscillator18/1 -> Product18/2
  Raised Cosine Transmit Filter9/1 -> Memoryless Nonlinearity8/1
  AWGN Channel3/1 -> Product15/1
  Raised Cosine Receive Filter6/1 -> AGC4/1
  Integer to Bit Converter13/1 -> Find Delay3/2, Error Rate Calculation6/2
  DVBS-APSK Demodulator Baseband6/1 -> Integer to Bit Converter13/1
  AGC4/1 -> MLSE Equalizer1/1, Modulated Constellation7/3
  AGC7/1 -> MLSE Equalizer2/1, Modulated Constellation9/3

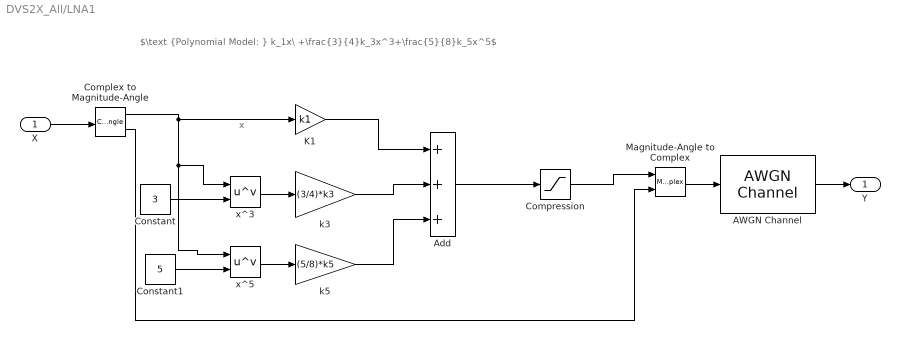
== system DVS2X_All/LNA1 ==
  note: x
  note: $\text {Polynomial Model: } k_1x\ +\frac{3}{4}k_3x^3+\frac{5}{8}k_5x^5$
  "X " : Inport
  AWGN Channel : commchan3/AWGN Channel  InputProcessing=Columns as channels (frame based)  seed=67  noiseMode="Signal to noise ratio  (Eb/No)"  EbNodB=23  EsNodB=10  SNRdB=10  bitsPerSym=4  Ps=1  Tsym=1e-6  variance=1
  Add : Sum  Inputs=+++
  Complex to Magnitude-Angle : ComplexToMagnitudeAngle
  "Compression " : Saturate  UpperLimit=2/3*vip3  LowerLimit=-1000
  Constant : Constant  Value=3
  Constant1 : Constant  Value=5
  K1 : Gain  Gain=k1
  Magnitude-Angle to Complex : MagnitudeAngleToComplex
  k3 : Gain  Gain=(3/4)*k3
  k5 : Gain  Gain=(5/8)*k5
  x^3 : Math  Operator=pow  SaturateOnIntegerOverflow=on
  x^5 : Math  Operator=pow  SaturateOnIntegerOverflow=on
  "Y " : Outport
  wires:
  Add/1 -> "Compression "/1
  Constant/1 -> x^3/2
  x^3/1 -> k3/1
  Constant1/1 -> x^5/2
  x^5/1 -> k5/1
  K1/1 -> Add/1
  k3/1 -> Add/2
  k5/1 -> Add/3
  "X "/1 -> Complex to Magnitude-Angle/1
  Complex to Magnitude-Angle/1 -> x^5/1, x^3/1, K1/1
  Complex to Magnitude-Angle/2 -> Magnitude-Angle to Complex/2
  "Compression "/1 -> Magnitude-Angle to Complex/1
  Magnitude-Angle to Complex/1 -> AWGN Channel/1
  AWGN Channel/1 -> "Y "/1

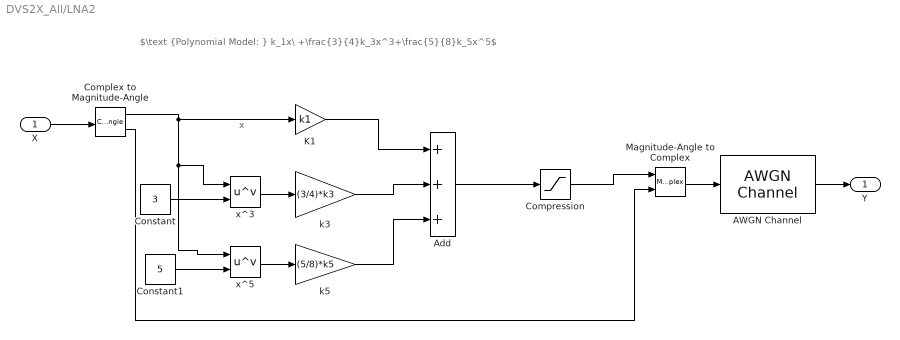
== system DVS2X_All/LNA2 ==
  note: x
  note: $\text {Polynomial Model: } k_1x\ +\frac{3}{4}k_3x^3+\frac{5}{8}k_5x^5$
  "X " : Inport
  AWGN Channel : commchan3/AWGN Channel  InputProcessing=Columns as channels (frame based)  seed=67  noiseMode="Signal to noise ratio  (Eb/No)"  EbNodB=23  EsNodB=10  SNRdB=10  bitsPerSym=4  Ps=1  Tsym=1e-6  variance=1
  Add : Sum  Inputs=+++
  Complex to Magnitude-Angle : ComplexToMagnitudeAngle
  "Compression " : Saturate  UpperLimit=2/3*vip3  LowerLimit=-1000
  Constant : Constant  Value=3
  Constant1 : Constant  Value=5
  K1 : Gain  Gain=k1
  Magnitude-Angle to Complex : MagnitudeAngleToComplex
  k3 : Gain  Gain=(3/4)*k3
  k5 : Gain  Gain=(5/8)*k5
  x^3 : Math  Operator=pow  SaturateOnIntegerOverflow=on
  x^5 : Math  Operator=pow  SaturateOnIntegerOverflow=on
  "Y " : Outport
  wires:
  Add/1 -> "Compression "/1
  Constant/1 -> x^3/2
  x^3/1 -> k3/1
  Constant1/1 -> x^5/2
  x^5/1 -> k5/1
  K1/1 -> Add/1
  k3/1 -> Add/2
  k5/1 -> Add/3
  "X "/1 -> Complex to Magnitude-Angle/1
  Complex to Magnitude-Angle/1 -> x^5/1, x^3/1, K1/1
  Complex to Magnitude-Angle/2 -> Magnitude-Angle to Complex/2
  "Compression "/1 -> Magnitude-Angle to Complex/1
  Magnitude-Angle to Complex/1 -> AWGN Channel/1
  AWGN Channel/1 -> "Y "/1

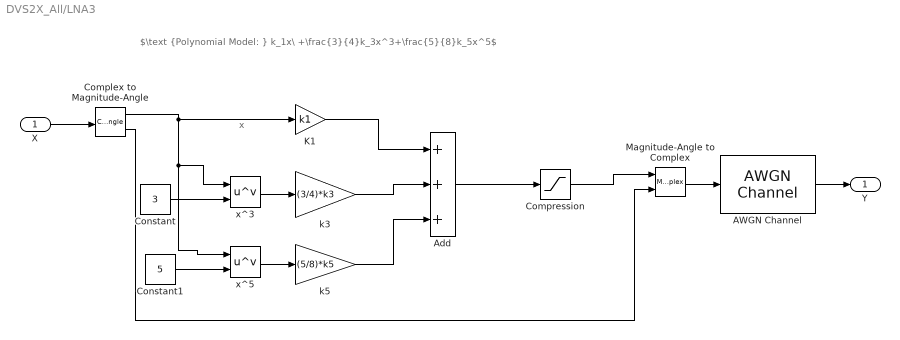
== system DVS2X_All/LNA3 ==
  note: x
  note: $\text {Polynomial Model: } k_1x\ +\frac{3}{4}k_3x^3+\frac{5}{8}k_5x^5$
  "X " : Inport
  AWGN Channel : commchan3/AWGN Channel  InputProcessing=Columns as channels (frame based)  seed=67  noiseMode="Signal to noise ratio  (Eb/No)"  EbNodB=23  EsNodB=10  SNRdB=10  bitsPerSym=4  Ps=1  Tsym=1e-6  variance=1
  Add : Sum  Inputs=+++
  Complex to Magnitude-Angle : ComplexToMagnitudeAngle
  "Compression " : Saturate  UpperLimit=2/3*vip3  LowerLimit=-1000
  Constant : Constant  Value=3
  Constant1 : Constant  Value=5
  K1 : Gain  Gain=k1
  Magnitude-Angle to Complex : MagnitudeAngleToComplex
  k3 : Gain  Gain=(3/4)*k3
  k5 : Gain  Gain=(5/8)*k5
  x^3 : Math  Operator=pow  SaturateOnIntegerOverflow=on
  x^5 : Math  Operator=pow  SaturateOnIntegerOverflow=on
  "Y " : Outport
  wires:
  Add/1 -> "Compression "/1
  Constant/1 -> x^3/2
  x^3/1 -> k3/1
  Constant1/1 -> x^5/2
  x^5/1 -> k5/1
  K1/1 -> Add/1
  k3/1 -> Add/2
  k5/1 -> Add/3
  "X "/1 -> Complex to Magnitude-Angle/1
  Complex to Magnitude-Angle/1 -> x^5/1, x^3/1, K1/1
  Complex to Magnitude-Angle/2 -> Magnitude-Angle to Complex/2
  "Compression "/1 -> Magnitude-Angle to Complex/1
  Magnitude-Angle to Complex/1 -> AWGN Channel/1
  AWGN Channel/1 -> "Y "/1

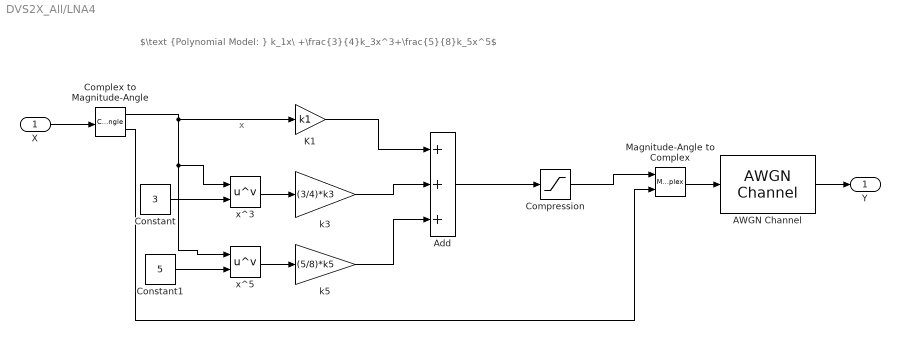
== system DVS2X_All/LNA4 ==
  note: x
  note: $\text {Polynomial Model: } k_1x\ +\frac{3}{4}k_3x^3+\frac{5}{8}k_5x^5$
  "X " : Inport
  AWGN Channel : commchan3/AWGN Channel  InputProcessing=Columns as channels (frame based)  seed=67  noiseMode="Signal to noise ratio  (Eb/No)"  EbNodB=23  EsNodB=10  SNRdB=10  bitsPerSym=4  Ps=1  Tsym=1e-6  variance=1
  Add : Sum  Inputs=+++
  Complex to Magnitude-Angle : ComplexToMagnitudeAngle
  "Compression " : Saturate  UpperLimit=2/3*vip3  LowerLimit=-1000
  Constant : Constant  Value=3
  Constant1 : Constant  Value=5
  K1 : Gain  Gain=k1
  Magnitude-Angle to Complex : MagnitudeAngleToComplex
  k3 : Gain  Gain=(3/4)*k3
  k5 : Gain  Gain=(5/8)*k5
  x^3 : Math  Operator=pow  SaturateOnIntegerOverflow=on
  x^5 : Math  Operator=pow  SaturateOnIntegerOverflow=on
  "Y " : Outport
  wires:
  Add/1 -> "Compression "/1
  Constant/1 -> x^3/2
  x^3/1 -> k3/1
  Constant1/1 -> x^5/2
  x^5/1 -> k5/1
  K1/1 -> Add/1
  k3/1 -> Add/2
  k5/1 -> Add/3
  "X "/1 -> Complex to Magnitude-Angle/1
  Complex to Magnitude-Angle/1 -> x^5/1, x^3/1, K1/1
  Complex to Magnitude-Angle/2 -> Magnitude-Angle to Complex/2
  "Compression "/1 -> Magnitude-Angle to Complex/1
  Magnitude-Angle to Complex/1 -> AWGN Channel/1
  AWGN Channel/1 -> "Y "/1

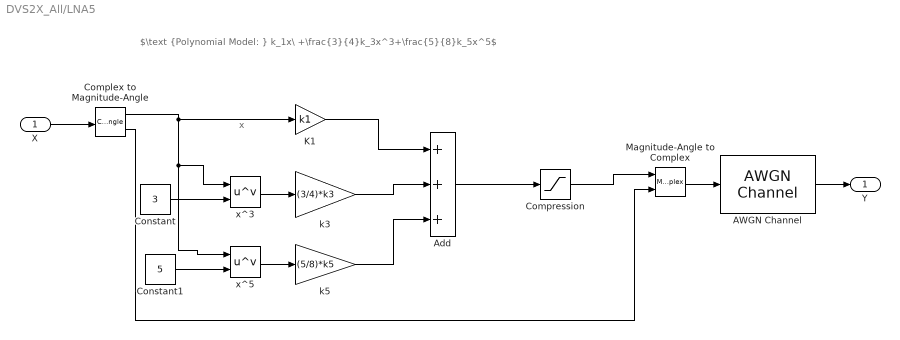
== system DVS2X_All/LNA5 ==
  note: x
  note: $\text {Polynomial Model: } k_1x\ +\frac{3}{4}k_3x^3+\frac{5}{8}k_5x^5$
  "X " : Inport
  AWGN Channel : commchan3/AWGN Channel  InputProcessing=Columns as channels (frame based)  seed=67  noiseMode="Signal to noise ratio  (Eb/No)"  EbNodB=50  EsNodB=10  SNRdB=10  bitsPerSym=4  Ps=1  Tsym=1e-6  variance=1
  Add : Sum  Inputs=+++
  Complex to Magnitude-Angle : ComplexToMagnitudeAngle
  "Compression " : Saturate  UpperLimit=2/3*vip3  LowerLimit=-1000
  Constant : Constant  Value=3
  Constant1 : Constant  Value=5
  K1 : Gain  Gain=k1
  Magnitude-Angle to Complex : MagnitudeAngleToComplex
  k3 : Gain  Gain=(3/4)*k3
  k5 : Gain  Gain=(5/8)*k5
  x^3 : Math  Operator=pow  SaturateOnIntegerOverflow=on
  x^5 : Math  Operator=pow  SaturateOnIntegerOverflow=on
  "Y " : Outport
  wires:
  Add/1 -> "Compression "/1
  Constant/1 -> x^3/2
  x^3/1 -> k3/1
  Constant1/1 -> x^5/2
  x^5/1 -> k5/1
  K1/1 -> Add/1
  k3/1 -> Add/2
  k5/1 -> Add/3
  "X "/1 -> Complex to Magnitude-Angle/1
  Complex to Magnitude-Angle/1 -> x^5/1, x^3/1, K1/1
  Complex to Magnitude-Angle/2 -> Magnitude-Angle to Complex/2
  "Compression "/1 -> Magnitude-Angle to Complex/1
  Magnitude-Angle to Complex/1 -> AWGN Channel/1
  AWGN Channel/1 -> "Y "/1

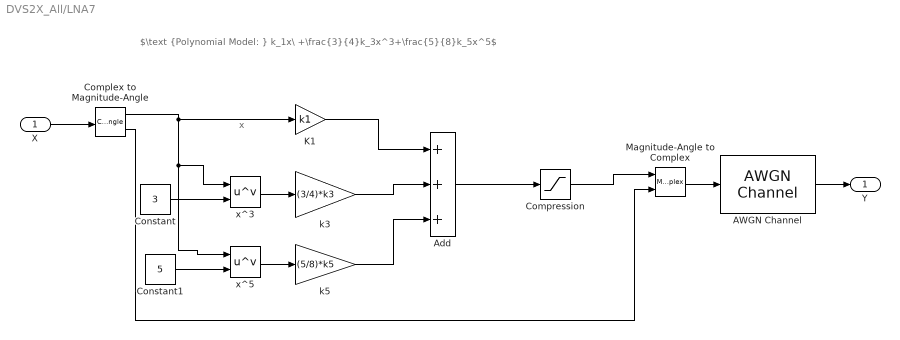
== system DVS2X_All/LNA7 ==
  note: x
  note: $\text {Polynomial Model: } k_1x\ +\frac{3}{4}k_3x^3+\frac{5}{8}k_5x^5$
  "X " : Inport
  AWGN Channel : commchan3/AWGN Channel  InputProcessing=Columns as channels (frame based)  seed=67  noiseMode="Signal to noise ratio  (Eb/No)"  EbNodB=23  EsNodB=10  SNRdB=10  bitsPerSym=4  Ps=1  Tsym=1e-6  variance=1
  Add : Sum  Inputs=+++
  Complex to Magnitude-Angle : ComplexToMagnitudeAngle
  "Compression " : Saturate  UpperLimit=2/3*vip3  LowerLimit=-1000
  Constant : Constant  Value=3
  Constant1 : Constant  Value=5
  K1 : Gain  Gain=k1
  Magnitude-Angle to Complex : MagnitudeAngleToComplex
  k3 : Gain  Gain=(3/4)*k3
  k5 : Gain  Gain=(5/8)*k5
  x^3 : Math  Operator=pow  SaturateOnIntegerOverflow=on
  x^5 : Math  Operator=pow  SaturateOnIntegerOverflow=on
  "Y " : Outport
  wires:
  Add/1 -> "Compression "/1
  Constant/1 -> x^3/2
  x^3/1 -> k3/1
  Constant1/1 -> x^5/2
  x^5/1 -> k5/1
  K1/1 -> Add/1
  k3/1 -> Add/2
  k5/1 -> Add/3
  "X "/1 -> Complex to Magnitude-Angle/1
  Complex to Magnitude-Angle/1 -> x^5/1, x^3/1, K1/1
  Complex to Magnitude-Angle/2 -> Magnitude-Angle to Complex/2
  "Compression "/1 -> Magnitude-Angle to Complex/1
  Magnitude-Angle to Complex/1 -> AWGN Channel/1
  AWGN Channel/1 -> "Y "/1
